simulink model "6DoF_V8_2024a_FULLY_WORKING_FG"  (R2024b)
settings: Solver=ode45  StartTime=0.0  StopTime=500  FixedStep=.01  MaxStep=.004  RelTol=1e-5  EnableMultiTasking=on
values from neighbouring files (symbols this model uses):
  ac = [0 0 0]    [Geom_6dof_V4_WITH_MAP.m]
  b = 33.4    [Geom_6dof_V4_WITH_MAP.m]
  bankrange = linspace(-pi,pi,100)    [Geom_6dof_V4_WITH_MAP.m]
  cbar = 5.7    [Geom_6dof_V4_WITH_MAP.m]
  cda2 = 0.33    [Geom_6dof_V4_WITH_MAP.m]
  cdo = 0.05    [Geom_6dof_V4_WITH_MAP.m]
  cg = [0 0 0]    [Geom_6dof_V4_WITH_MAP.m]
  cla = 4.44    [Geom_6dof_V4_WITH_MAP.m]
  cladot = 0    [Geom_6dof_V4_WITH_MAP.m]
  clb = -0.074    [Geom_6dof_V4_WITH_MAP.m]
  clda = -0.134    [Geom_6dof_V4_WITH_MAP.m]
  clde = 0.355    [Geom_6dof_V4_WITH_MAP.m]
  cldr = 0.107    [Geom_6dof_V4_WITH_MAP.m]
  clo = 0.41    [Geom_6dof_V4_WITH_MAP.m]
  clp = -0.410    (= -0.41)    [Geom_6dof_V4_WITH_MAP.m]
  clq = 3.8    [Geom_6dof_V4_WITH_MAP.m]
  clr = 0.107    [Geom_6dof_V4_WITH_MAP.m]
  cma = -0.683    [Geom_6dof_V4_WITH_MAP.m]
  cmadot = -4.36    [Geom_6dof_V4_WITH_MAP.m]
  cmde = -0.923    [Geom_6dof_V4_WITH_MAP.m]
  cmq = -9.96    [Geom_6dof_V4_WITH_MAP.m]
  cnb = 0.071    [Geom_6dof_V4_WITH_MAP.m]
  cnda = -0.0035    [Geom_6dof_V4_WITH_MAP.m]
  cndr = -0.072    [Geom_6dof_V4_WITH_MAP.m]
  cnp = -0.0575    [Geom_6dof_V4_WITH_MAP.m]
  cnr = -0.125    [Geom_6dof_V4_WITH_MAP.m]
  cyb = -0.564    [Geom_6dof_V4_WITH_MAP.m]
  cydr = 0.157    [Geom_6dof_V4_WITH_MAP.m]
  eng = [0 0 0]    [Geom_6dof_V4_WITH_MAP.m]
  initalt = 5000    [Geom_6dof_V4_WITH_MAP.m]
  initbank = 0    [Geom_6dof_V4_WITH_MAP.m]
  initeast = 0    [Geom_6dof_V4_WITH_MAP.m]
  inithead = 0    [Geom_6dof_V4_WITH_MAP.m]
  initnorth = 0    [Geom_6dof_V4_WITH_MAP.m]
  initp = 0    [Geom_6dof_V4_WITH_MAP.m]
  initpitch = initw/initu    (= -0.0287187462721)    [Geom_6dof_V4_WITH_MAP.m]
  initq = 0    [Geom_6dof_V4_WITH_MAP.m]
  initr = 0    [Geom_6dof_V4_WITH_MAP.m]
  initu = 226.333    [Geom_6dof_V4_WITH_MAP.m]
  initv = 0    [Geom_6dof_V4_WITH_MAP.m]
  initw = -6.5    [Geom_6dof_V4_WITH_MAP.m]
  jx = 1048    [Geom_6dof_V4_WITH_MAP.m]
  jxz = 0    [Geom_6dof_V4_WITH_MAP.m]
  jy = 3000    [Geom_6dof_V4_WITH_MAP.m]
  jz = 3500    [Geom_6dof_V4_WITH_MAP.m]
  sw = 184    [Geom_6dof_V4_WITH_MAP.m]
  weight = 2750    [Geom_6dof_V4_WITH_MAP.m]
  WP1 = [10000 10000 5000]    [Geom_6dof_V4_WITH_MAP.m]
  WP2 = [-10000 0 5500]    [Geom_6dof_V4_WITH_MAP.m]
  WP3 = [0 -10000 4500]    [Geom_6dof_V4_WITH_MAP.m]
libraries: slpidlib x10, simulink_extras x5, aerolibfltsims x2, aerolibanimutils x1, dspswit3 x1
(part 2 of 2)

== system 6DoF_V8_2024a_FULLY_WORKING_FG/Aircraft_Dynamics/Equations of motion numerical integration /Gravity Model ==
  Constant : Constant  Value=0
  Constant1 : Constant  Value=32.2
  Mux : Mux  Inputs=3
  Gravity : Outport
  wires:
  Constant/1 -> Mux/1, Mux/2
  Constant1/1 -> Mux/3
  Mux/1 -> Gravity/1

== system 6DoF_V8_2024a_FULLY_WORKING_FG/Aircraft_Dynamics/Equations of motion numerical integration /Inert-body ==
  Euler : Inport
  11 : Fcn  Expr=cos(u[2])*cos(u[3])
  12 : Fcn  Expr=-cos(u[1])*sin(u[3])+sin(u[1])*sin(u[2])*cos(u[3])
  13 : Fcn  Expr=sin(u[1])*sin(u[3])+cos(u[1])*sin(u[2])*cos(u[3])
  21 : Fcn  Expr=cos(u[2])*sin(u[3])
  22 : Fcn  Expr=cos(u[1])*cos(u[3]) + sin(u[1])*sin(u[2])*sin(u[3])
  23 : Fcn  Expr=-sin(u[1])*cos(u[3])+cos(u[1])*sin(u[2])*sin(u[3])
  31 : Fcn  Expr=-sin(u[2])
  32 : Fcn  Expr=sin(u[1]) * cos(u[2])
  33 : Fcn  Expr=cos(u[1])*cos(u[2])
  Matrix Concatenation : Concatenate  NumInputs=3  Mode=Multidimensional array
  Matrix Concatenation1 : Concatenate  NumInputs=3  Mode=Multidimensional array
  Matrix Concatenation2 : Concatenate  NumInputs=3  Mode=Multidimensional array
  Matrix Concatenation3 : Concatenate  NumInputs=3  Mode=Multidimensional array  ConcatenateDimension=2
  NEDtoBC : Outport
  wires:
  Euler/1 -> 11/1, 12/1, 13/1, 21/1, 22/1, 23/1, 31/1, 33/1, 32/1
  12/1 -> Matrix Concatenation/2
  11/1 -> Matrix Concatenation/1
  13/1 -> Matrix Concatenation/3
  22/1 -> Matrix Concatenation1/2
  21/1 -> Matrix Concatenation1/1
  23/1 -> Matrix Concatenation1/3
  32/1 -> Matrix Concatenation2/2
  31/1 -> Matrix Concatenation2/1
  33/1 -> Matrix Concatenation2/3
  Matrix Concatenation1/1 -> Matrix Concatenation3/2
  Matrix Concatenation/1 -> Matrix Concatenation3/1
  Matrix Concatenation2/1 -> Matrix Concatenation3/3
  Matrix Concatenation3/1 -> NEDtoBC/1

== system 6DoF_V8_2024a_FULLY_WORKING_FG/Aircraft_Dynamics/Equations of motion numerical integration /Kinematic Equiations ==
  note: 1  p
      | 2  q
      | 3  r
      | 4  bank
      | 5 pitch
      | 6 Yaw
  Rates : Inport
  2pi Bound : Subsystem  mask(2pi bound){}
      mask help: Bounds the input angle to [0, 2pi]. When 0 bound is exceeded the output wraps back to 2pi; when the 2pi bound is exceeded the output wraps back to 0.
      mask Help:
      | Bounds the input angle to [0, 2pi]. When 0 bound is exceeded the output wraps back to 2pi; when the 2pi bound is exceeded the output wraps back to 0.
      | <P><B>Input:</B> any angle in radians, from -Inf to Inf;</P>
      | <P><B>Output:</B> an angle in radians between zero and 2pi.</P>
  Demux : Demux  Outputs=3
      settings: DisplayOption=none
  Demux1 : Demux  Outputs=3
      settings: DisplayOption=none
  Demux2 : Demux  Outputs=3
      settings: DisplayOption=none
  Mux : Mux  Inputs=6
  Mux1 : Mux  Inputs=3
  Mux2 : Mux  Inputs=3
  Yaw rate : Fcn  Expr=(u[2] * sin(u[4]) + u[3] * cos(u[4]))/cos(u[5])
  bank : Integrator  InitialCondition=initbank
  heading : Integrator  InitialCondition=inithead
  pi Bound : Subsystem  mask(pi bound){}
      mask help: Bounds the input angle to [-pi, pi]. When -pi bound is exceeded the output wraps back to pi; when the pi bound is exceeded the output wraps back to -pi.
      mask Help:
      | Bounds the input angle to [-pi, pi]. When -pi bound is exceeded the output wraps back to pi; when the pi bound is exceeded the output wraps back to -pi.
      | <P><B>Input:</B> any angle in radians, from -Inf to Inf;</P>
      | <P><B>Output:</B> an angle in radians between -pi and pi.</P>
  pi Bound1 : Subsystem  mask(pi bound){}
      mask help: Bounds the input angle to [-pi, pi]. When -pi bound is exceeded the output wraps back to pi; when the pi bound is exceeded the output wraps back to -pi.
      mask Help:
      | Bounds the input angle to [-pi, pi]. When -pi bound is exceeded the output wraps back to pi; when the pi bound is exceeded the output wraps back to -pi.
      | <P><B>Input:</B> any angle in radians, from -Inf to Inf;</P>
      | <P><B>Output:</B> an angle in radians between -pi and pi.</P>
  pitch : Integrator  InitialCondition=initpitch
  pitch rate : Fcn  Expr=u[2] *cos(u[4]) - u[3] * sin(u[4])
  roll rate : Fcn  Expr=u[1] + tan(u[5])*(u[2]*sin(u[4])+u[3]*cos(u[4]))
  Euler angles : Outport
  wires:
  Rates/1 -> Demux/1
  Demux/2 -> Mux/2
  Demux/3 -> Mux/3
  Demux1/1 -> Mux/4
  Demux1/2 -> Mux/5
  Demux1/3 -> Mux/6
  Demux/1 -> Mux/1
  Mux/1 -> roll rate/1, Yaw rate/1, pitch rate/1
  Demux2/3 -> 2pi Bound/1(In)
  Demux2/2 -> pi Bound/1(In)
  Demux2/1 -> pi Bound1/1(In)
  Mux2/1 -> Euler angles/1
  pi Bound/1(Out) -> Mux2/2
  pi Bound1/1(Out) -> Mux2/1
  2pi Bound/1(Out) -> Mux2/3
  pitch rate/1 -> pitch/1
  roll rate/1 -> bank/1
  Yaw rate/1 -> heading/1
  bank/1 -> Mux1/1
  pitch/1 -> Mux1/2
  heading/1 -> Mux1/3
  Mux1/1 -> Demux2/1, Demux1/1

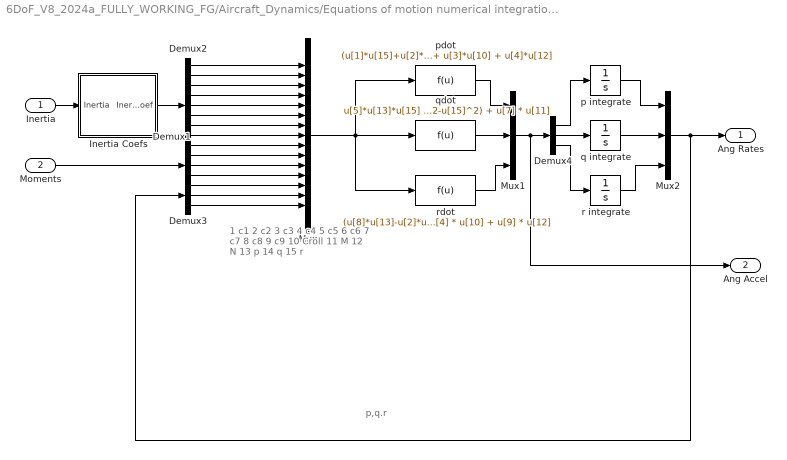
== system 6DoF_V8_2024a_FULLY_WORKING_FG/Aircraft_Dynamics/Equations of motion numerical integration /Moment Equations ==
  note: 1   c1
      | 2   c2
      | 3   c3
      | 4  c4
      | 5  c5
      | 6  c6
      | 7  c7
      | 8  c8
      | 9  c9
      | 10 Croll
      | 11  M
      | 12  N
      | 13  p
      | 14  q
      | 15  r
  note: p,q.r
  Inertia : Inport
  Moments : Inport  Port=2
  Demux1 : Demux  Outputs=3
      settings: DisplayOption=none
  Demux2 : Demux  Outputs=9
      settings: DisplayOption=none
  Demux3 : Demux  Outputs=3
      settings: DisplayOption=none
  Demux4 : Demux  Outputs=3
      settings: DisplayOption=none
  Inertia Coefs : Subsystem
  Mux : Mux  Inputs=15
  Mux1 : Mux  Inputs=3
  Mux2 : Mux  Inputs=3
  p integrate : Integrator  InitialCondition=initp
  pdot : Fcn  Expr=(u[1]*u[15]+u[2]*u[13])*u[14] + u[3]*u[10] + u[4]*u[12]
  q integrate : Integrator  InitialCondition=initq
  qdot : Fcn  Expr=u[5]*u[13]*u[15] - u[6]*(u[13]^2-u[15]^2) + u[7] * u[11]
  r integrate : Integrator  InitialCondition=initr
  rdot : Fcn  Expr=(u[8]*u[13]-u[2]*u[15]) * u[14] + u[4] * u[10] + u[9] * u[12]
  Ang Rates : Outport
  Ang Accel : Outport  Port=2
  wires:
  Inertia/1 -> Inertia Coefs/1(Inertia)
  Moments/1 -> Demux1/1
  Inertia Coefs/1(Iner Coef) -> Demux2/1
  Demux2/1 -> Mux/1
  Demux2/2 -> Mux/2
  Demux2/3 -> Mux/3
  Demux2/4 -> Mux/4
  Demux2/5 -> Mux/5
  Demux2/6 -> Mux/6
  Demux2/7 -> Mux/7
  Demux2/8 -> Mux/8
  Demux2/9 -> Mux/9
  Demux1/1 -> Mux/10
  Demux1/2 -> Mux/11
  Demux1/3 -> Mux/12
  Demux3/1 -> Mux/13
  Demux3/2 -> Mux/14
  Demux3/3 -> Mux/15
  Mux/1 -> pdot/1, qdot/1, rdot/1
  qdot/1 -> Mux1/2
  pdot/1 -> Mux1/1
  rdot/1 -> Mux1/3
  Mux1/1 -> Ang Accel/1, Demux4/1
  Demux4/1 -> p integrate/1
  Demux4/2 -> q integrate/1
  Demux4/3 -> r integrate/1
  Mux2/1 -> Ang Rates/1, Demux3/1
  p integrate/1 -> Mux2/1
  q integrate/1 -> Mux2/2
  r integrate/1 -> Mux2/3

== system 6DoF_V8_2024a_FULLY_WORKING_FG/Aircraft_Dynamics/Linear Acc and Moments/Cross Prod Moment due Leng ==
  Vec 1 : Inport
  Vec 2 : Inport  Port=2
  Check prob not zero : Constant  Value=0
  Demux : Demux  Outputs=3
      settings: DisplayOption=none
  J axis : Fcn  Expr=u[4]*u[3] - u[6]*u[1]
  Mux : Mux  Inputs=6
  Mux1 : Mux  Inputs=3
  i axis : Fcn  Expr=u[6]*u[2] - u[5]*u[3]
  k axis : Fcn  Expr=u[5]*u[1] - u[4]*u[2]
  X Prod : Outport
  wires:
  Vec 2/1 -> Mux/4
  Vec 1/1 -> Demux/1
  Demux/1 -> Mux/1
  Check prob not zero/1 -> Mux/5, Mux/6
  Demux/3 -> Mux/3
  Demux/2 -> Mux/2
  Mux/1 -> i axis/1, J axis/1, k axis/1
  J axis/1 -> Mux1/2
  i axis/1 -> Mux1/1
  k axis/1 -> Mux1/3
  Mux1/1 -> X Prod/1

== system 6DoF_V8_2024a_FULLY_WORKING_FG/Aircraft_Dynamics/Linear Acc and Moments/Cross Prod Moment due to Aero ==
  Vec 1 : Inport
  Vec 2 : Inport  Port=2
  Demux : Demux  Outputs=3
      settings: DisplayOption=none
  Demux1 : Demux  Outputs=3
      settings: DisplayOption=none
  J axis : Fcn  Expr=u[4]*u[3] - u[6]*u[1]
  Mux : Mux  Inputs=6
  Mux1 : Mux  Inputs=3
  i axis : Fcn  Expr=u[6]*u[2] - u[5]*u[3]
  k axis : Fcn  Expr=u[5]*u[1] - u[4]*u[2]
  X Prod : Outport
  wires:
  Vec 2/1 -> Demux1/1
  Vec 1/1 -> Demux/1
  Demux/1 -> Mux/1
  Demux1/3 -> Mux/6
  Demux1/2 -> Mux/5
  Demux1/1 -> Mux/4
  Demux/3 -> Mux/3
  Demux/2 -> Mux/2
  Mux/1 -> i axis/1, J axis/1, k axis/1
  J axis/1 -> Mux1/2
  i axis/1 -> Mux1/1
  k axis/1 -> Mux1/3
  Mux1/1 -> X Prod/1

== system 6DoF_V8_2024a_FULLY_WORKING_FG/Waypoint Calc/Altitude Hold Autopilot/Climb ==
  R/C : Inport
  Action Port : ActionPort  ActionPortLabel=if(u1 < -100)
  PID Controller : slpidlib/PID Controller  Controller=PI  Form=Parallel  TimeDomain=Continuous-time  UseExternalTs=off  SampleTime=-1  IntegratorMethod=Forward Euler  FilterMethod=Forward Euler  ControllerParametersSource=internal  P=-9.44462319155585e-06  I=-9.44462319155585e-06  UseKiTs=off  D=0  UseExternalDerivativeSource=off  N=100  UseFilter=on  TunerSelectOption=Transfer Function Based (PID Tuner App)  InitialConditionSource=internal  InitialConditionForIntegrator=0  InitialConditionForFilter=0  DifferentiatorICPrevScaledInput=0  ExternalReset=none  TrackingMode=off  Kt=1  LimitOutput=off  SatLimitsSource=internal  UpperSaturationLimit=inf  LowerSaturationLimit=-inf  LinearizeAsGain=on  AntiWindupMode=none  Kb=1  LimitIntegrator=off  UpperIntegratorSaturationLimit=inf  LowerIntegratorSaturationLimit=-inf  POutMin=[]  POutMax=[]  IOutMin=[]  IOutMax=[]  DOutMin=[]  DOutMax=[]  NOutMin=[]  NOutMax=[]  SumOutMin=[]  SumOutMax=[]  SaturationOutMin=[]  SaturationOutMax=[]  PParamMin=[]  PParamMax=[]  IParamMin=[]  IParamMax=[]  DParamMin=[]  DParamMax=[]  NParamMin=[]  NParamMax=[]  KbParamMin=[]  KbParamMax=[]  KtParamMin=[]  KtParamMax=[]  KbOutMin=[]  KbOutMax=[]  KtOutMin=[]  KtOutMax=[]  IntegratorOutMin=[]  IntegratorOutMax=[]  FilterOutMin=[]  FilterOutMax=[]  SumI1OutMin=[]  SumI1OutMax=[]  SumI2OutMin=[]  SumI2OutMax=[]  SumI3OutMin=[]  SumI3OutMax=[]  SumI4OutMin=[]  SumI4OutMax=[]  SumDOutMin=[]  SumDOutMax=[]  DifferentiatorOutMin=[]  DifferentiatorOutMax=[]  FilterDiffOutCoefMin=[]  FilterDiffOutCoefMax=[]  ReciprocalOutMin=[]  ReciprocalOutMax=[]  SumDenOutMin=[]  SumDenOutMax=[]  SumNumOutMin=[]  SumNumOutMax=[]  DivideOutMin=[]  DivideOutMax=[]  UdiffTsProdOutMin=[]  UdiffTsProdOutMax=[]  NTsProdOutMin=[]  NTsProdOutMax=[]  UintegralTsProdOutMin=[]  UintegralTsProdOutMax=[]  UngainTsProdOutMin=[]  UngainTsProdOutMax=[]  ClampingZeroOutDataTypeStr=Inherit: Inherit via back propagation  ClampingZeroOutMin=[]  ClampingZeroOutMax=[]  FilterDenConstantOutDataTypeStr=Inherit: Inherit via back propagation  FilterDenConstantOutMin=[]  FilterDenConstantOutMax=[]  PCopyOutDataTypeStr=Inherit: Inherit via back propagation  PCopyOutMin=[]  PCopyOutMax=[]  NCopyOutDataTypeStr=Inherit: Inherit via back propagation  NCopyOutMin=[]  NCopyOutMax=[]  IntegratorContinuousStateAttributes=''  IntegratorStateMustResolveToSignalObject=off  IntegratorRTWStateStorageClass=Auto  FilterContinuousStateAttributes=''  FilterStateMustResolveToSignalObject=off  FilterRTWStateStorageClass=Auto  ParallelPVariant=InternalParameters  IdealPVariant=Disabled  IVariant=InternalParameters  DVariant=Disabled  IntegratorVariant=Continuous  SatVariant=Disabled  AWVariant=Passthrough  PCopyVariant=Disabled  TRVariant=Disabled  FdbkBlocksVariant=Forward  IdealPFdbkVariant=Disabled  SatFdbkVariant=Disabled  DerivativeFilterVariant=Disabled  NVariant=Disabled  NCopyVariant=Disabled_SignalSpec  FilterICVariant=Disabled  IntegratorICVariant=InternalICs  ExternalResetVariant=Disabled  TRSumVariant=Passthrough  SumFdbkVariant=Disabled  SumVariant=Sum_PI  TsampFilterVariant=InternalTs  TsampNgainVariant=Passthrough  TsampIntegralVariant=Disabled_SignalSpec  ExternalSaturationOutDataTypeStr=Inherit: Same as second input  DerivativeSourceVariant=Disabled  PreIntVariant=InternalPreInt
  PID Controller1 : slpidlib/PID Controller  Controller=PI  Form=Parallel  TimeDomain=Continuous-time  UseExternalTs=off  SampleTime=-1  IntegratorMethod=Forward Euler  FilterMethod=Forward Euler  ControllerParametersSource=internal  P=-0.000713863552295223  I=-0.000143178740792475  UseKiTs=off  D=0  UseExternalDerivativeSource=off  N=100  UseFilter=on  TunerSelectOption=Transfer Function Based (PID Tuner App)  InitialConditionSource=internal  InitialConditionForIntegrator=0  InitialConditionForFilter=0  DifferentiatorICPrevScaledInput=0  ExternalReset=none  TrackingMode=off  Kt=1  LimitOutput=off  SatLimitsSource=internal  UpperSaturationLimit=inf  LowerSaturationLimit=-inf  LinearizeAsGain=on  AntiWindupMode=none  Kb=1  LimitIntegrator=off  UpperIntegratorSaturationLimit=inf  LowerIntegratorSaturationLimit=-inf  POutMin=[]  POutMax=[]  IOutMin=[]  IOutMax=[]  DOutMin=[]  DOutMax=[]  NOutMin=[]  NOutMax=[]  SumOutMin=[]  SumOutMax=[]  SaturationOutMin=[]  SaturationOutMax=[]  PParamMin=[]  PParamMax=[]  IParamMin=[]  IParamMax=[]  DParamMin=[]  DParamMax=[]  NParamMin=[]  NParamMax=[]  KbParamMin=[]  KbParamMax=[]  KtParamMin=[]  KtParamMax=[]  KbOutMin=[]  KbOutMax=[]  KtOutMin=[]  KtOutMax=[]  IntegratorOutMin=[]  IntegratorOutMax=[]  FilterOutMin=[]  FilterOutMax=[]  SumI1OutMin=[]  SumI1OutMax=[]  SumI2OutMin=[]  SumI2OutMax=[]  SumI3OutMin=[]  SumI3OutMax=[]  SumI4OutMin=[]  SumI4OutMax=[]  SumDOutMin=[]  SumDOutMax=[]  DifferentiatorOutMin=[]  DifferentiatorOutMax=[]  FilterDiffOutCoefMin=[]  FilterDiffOutCoefMax=[]  ReciprocalOutMin=[]  ReciprocalOutMax=[]  SumDenOutMin=[]  SumDenOutMax=[]  SumNumOutMin=[]  SumNumOutMax=[]  DivideOutMin=[]  DivideOutMax=[]  UdiffTsProdOutMin=[]  UdiffTsProdOutMax=[]  NTsProdOutMin=[]  NTsProdOutMax=[]  UintegralTsProdOutMin=[]  UintegralTsProdOutMax=[]  UngainTsProdOutMin=[]  UngainTsProdOutMax=[]  ClampingZeroOutDataTypeStr=Inherit: Inherit via back propagation  ClampingZeroOutMin=[]  ClampingZeroOutMax=[]  FilterDenConstantOutDataTypeStr=Inherit: Inherit via back propagation  FilterDenConstantOutMin=[]  FilterDenConstantOutMax=[]  PCopyOutDataTypeStr=Inherit: Inherit via back propagation  PCopyOutMin=[]  PCopyOutMax=[]  NCopyOutDataTypeStr=Inherit: Inherit via back propagation  NCopyOutMin=[]  NCopyOutMax=[]  IntegratorContinuousStateAttributes=''  IntegratorStateMustResolveToSignalObject=off  IntegratorRTWStateStorageClass=Auto  FilterContinuousStateAttributes=''  FilterStateMustResolveToSignalObject=off  FilterRTWStateStorageClass=Auto  ParallelPVariant=InternalParameters  IdealPVariant=Disabled  IVariant=InternalParameters  DVariant=Disabled  IntegratorVariant=Continuous  SatVariant=Disabled  AWVariant=Passthrough  PCopyVariant=Disabled  TRVariant=Disabled  FdbkBlocksVariant=Forward  IdealPFdbkVariant=Disabled  SatFdbkVariant=Disabled  DerivativeFilterVariant=Disabled  NVariant=Disabled  NCopyVariant=Disabled_SignalSpec  FilterICVariant=Disabled  IntegratorICVariant=InternalICs  ExternalResetVariant=Disabled  TRSumVariant=Passthrough  SumFdbkVariant=Disabled  SumVariant=Sum_PI  TsampFilterVariant=InternalTs  TsampNgainVariant=Passthrough  TsampIntegralVariant=Disabled_SignalSpec  ExternalSaturationOutDataTypeStr=Inherit: Same as second input  DerivativeSourceVariant=Disabled  PreIntVariant=InternalPreInt
  R/C_CMD : Constant  Value=12
  R/C_CMD1 : Constant
  Sum : Sum  Inputs=|+-
  del_e : Outport
  Debug : Outport  Port=2
  wires:
  R/C/1 -> Sum/1
  R/C_CMD/1 -> Sum/2
  R/C_CMD1/1 -> Debug/1
  Sum/1 -> PID Controller1/1
  PID Controller1/1 -> del_e/1

== system 6DoF_V8_2024a_FULLY_WORKING_FG/Waypoint Calc/Altitude Hold Autopilot/Descent ==
  R/C : Inport
  Action Port : ActionPort  ActionPortLabel=elseif(u1 > 100)
  Gain : Gain
  PID Controller : slpidlib/PID Controller  Controller=PI  Form=Parallel  TimeDomain=Continuous-time  UseExternalTs=off  SampleTime=-1  IntegratorMethod=Forward Euler  FilterMethod=Forward Euler  ControllerParametersSource=internal  P=-9.44462319155585e-06  I=-9.44462319155585e-06  UseKiTs=off  D=0  UseExternalDerivativeSource=off  N=100  UseFilter=on  TunerSelectOption=Transfer Function Based (PID Tuner App)  InitialConditionSource=internal  InitialConditionForIntegrator=0  InitialConditionForFilter=0  DifferentiatorICPrevScaledInput=0  ExternalReset=none  TrackingMode=off  Kt=1  LimitOutput=off  SatLimitsSource=internal  UpperSaturationLimit=inf  LowerSaturationLimit=-inf  LinearizeAsGain=on  AntiWindupMode=none  Kb=1  LimitIntegrator=off  UpperIntegratorSaturationLimit=inf  LowerIntegratorSaturationLimit=-inf  POutMin=[]  POutMax=[]  IOutMin=[]  IOutMax=[]  DOutMin=[]  DOutMax=[]  NOutMin=[]  NOutMax=[]  SumOutMin=[]  SumOutMax=[]  SaturationOutMin=[]  SaturationOutMax=[]  PParamMin=[]  PParamMax=[]  IParamMin=[]  IParamMax=[]  DParamMin=[]  DParamMax=[]  NParamMin=[]  NParamMax=[]  KbParamMin=[]  KbParamMax=[]  KtParamMin=[]  KtParamMax=[]  KbOutMin=[]  KbOutMax=[]  KtOutMin=[]  KtOutMax=[]  IntegratorOutMin=[]  IntegratorOutMax=[]  FilterOutMin=[]  FilterOutMax=[]  SumI1OutMin=[]  SumI1OutMax=[]  SumI2OutMin=[]  SumI2OutMax=[]  SumI3OutMin=[]  SumI3OutMax=[]  SumI4OutMin=[]  SumI4OutMax=[]  SumDOutMin=[]  SumDOutMax=[]  DifferentiatorOutMin=[]  DifferentiatorOutMax=[]  FilterDiffOutCoefMin=[]  FilterDiffOutCoefMax=[]  ReciprocalOutMin=[]  ReciprocalOutMax=[]  SumDenOutMin=[]  SumDenOutMax=[]  SumNumOutMin=[]  SumNumOutMax=[]  DivideOutMin=[]  DivideOutMax=[]  UdiffTsProdOutMin=[]  UdiffTsProdOutMax=[]  NTsProdOutMin=[]  NTsProdOutMax=[]  UintegralTsProdOutMin=[]  UintegralTsProdOutMax=[]  UngainTsProdOutMin=[]  UngainTsProdOutMax=[]  ClampingZeroOutDataTypeStr=Inherit: Inherit via back propagation  ClampingZeroOutMin=[]  ClampingZeroOutMax=[]  FilterDenConstantOutDataTypeStr=Inherit: Inherit via back propagation  FilterDenConstantOutMin=[]  FilterDenConstantOutMax=[]  PCopyOutDataTypeStr=Inherit: Inherit via back propagation  PCopyOutMin=[]  PCopyOutMax=[]  NCopyOutDataTypeStr=Inherit: Inherit via back propagation  NCopyOutMin=[]  NCopyOutMax=[]  IntegratorContinuousStateAttributes=''  IntegratorStateMustResolveToSignalObject=off  IntegratorRTWStateStorageClass=Auto  FilterContinuousStateAttributes=''  FilterStateMustResolveToSignalObject=off  FilterRTWStateStorageClass=Auto  ParallelPVariant=InternalParameters  IdealPVariant=Disabled  IVariant=InternalParameters  DVariant=Disabled  IntegratorVariant=Continuous  SatVariant=Disabled  AWVariant=Passthrough  PCopyVariant=Disabled  TRVariant=Disabled  FdbkBlocksVariant=Forward  IdealPFdbkVariant=Disabled  SatFdbkVariant=Disabled  DerivativeFilterVariant=Disabled  NVariant=Disabled  NCopyVariant=Disabled_SignalSpec  FilterICVariant=Disabled  IntegratorICVariant=InternalICs  ExternalResetVariant=Disabled  TRSumVariant=Passthrough  SumFdbkVariant=Disabled  SumVariant=Sum_PI  TsampFilterVariant=InternalTs  TsampNgainVariant=Passthrough  TsampIntegralVariant=Disabled_SignalSpec  ExternalSaturationOutDataTypeStr=Inherit: Same as second input  DerivativeSourceVariant=Disabled  PreIntVariant=InternalPreInt
  PID Controller1 : slpidlib/PID Controller  Controller=PI  Form=Parallel  TimeDomain=Continuous-time  UseExternalTs=off  SampleTime=-1  IntegratorMethod=Forward Euler  FilterMethod=Forward Euler  ControllerParametersSource=internal  P=-0.000713863552295223  I=-0.000143178740792475  UseKiTs=off  D=0  UseExternalDerivativeSource=off  N=100  UseFilter=on  TunerSelectOption=Transfer Function Based (PID Tuner App)  InitialConditionSource=internal  InitialConditionForIntegrator=0  InitialConditionForFilter=0  DifferentiatorICPrevScaledInput=0  ExternalReset=none  TrackingMode=off  Kt=1  LimitOutput=off  SatLimitsSource=internal  UpperSaturationLimit=inf  LowerSaturationLimit=-inf  LinearizeAsGain=on  AntiWindupMode=none  Kb=1  LimitIntegrator=off  UpperIntegratorSaturationLimit=inf  LowerIntegratorSaturationLimit=-inf  POutMin=[]  POutMax=[]  IOutMin=[]  IOutMax=[]  DOutMin=[]  DOutMax=[]  NOutMin=[]  NOutMax=[]  SumOutMin=[]  SumOutMax=[]  SaturationOutMin=[]  SaturationOutMax=[]  PParamMin=[]  PParamMax=[]  IParamMin=[]  IParamMax=[]  DParamMin=[]  DParamMax=[]  NParamMin=[]  NParamMax=[]  KbParamMin=[]  KbParamMax=[]  KtParamMin=[]  KtParamMax=[]  KbOutMin=[]  KbOutMax=[]  KtOutMin=[]  KtOutMax=[]  IntegratorOutMin=[]  IntegratorOutMax=[]  FilterOutMin=[]  FilterOutMax=[]  SumI1OutMin=[]  SumI1OutMax=[]  SumI2OutMin=[]  SumI2OutMax=[]  SumI3OutMin=[]  SumI3OutMax=[]  SumI4OutMin=[]  SumI4OutMax=[]  SumDOutMin=[]  SumDOutMax=[]  DifferentiatorOutMin=[]  DifferentiatorOutMax=[]  FilterDiffOutCoefMin=[]  FilterDiffOutCoefMax=[]  ReciprocalOutMin=[]  ReciprocalOutMax=[]  SumDenOutMin=[]  SumDenOutMax=[]  SumNumOutMin=[]  SumNumOutMax=[]  DivideOutMin=[]  DivideOutMax=[]  UdiffTsProdOutMin=[]  UdiffTsProdOutMax=[]  NTsProdOutMin=[]  NTsProdOutMax=[]  UintegralTsProdOutMin=[]  UintegralTsProdOutMax=[]  UngainTsProdOutMin=[]  UngainTsProdOutMax=[]  ClampingZeroOutDataTypeStr=Inherit: Inherit via back propagation  ClampingZeroOutMin=[]  ClampingZeroOutMax=[]  FilterDenConstantOutDataTypeStr=Inherit: Inherit via back propagation  FilterDenConstantOutMin=[]  FilterDenConstantOutMax=[]  PCopyOutDataTypeStr=Inherit: Inherit via back propagation  PCopyOutMin=[]  PCopyOutMax=[]  NCopyOutDataTypeStr=Inherit: Inherit via back propagation  NCopyOutMin=[]  NCopyOutMax=[]  IntegratorContinuousStateAttributes=''  IntegratorStateMustResolveToSignalObject=off  IntegratorRTWStateStorageClass=Auto  FilterContinuousStateAttributes=''  FilterStateMustResolveToSignalObject=off  FilterRTWStateStorageClass=Auto  ParallelPVariant=InternalParameters  IdealPVariant=Disabled  IVariant=InternalParameters  DVariant=Disabled  IntegratorVariant=Continuous  SatVariant=Disabled  AWVariant=Passthrough  PCopyVariant=Disabled  TRVariant=Disabled  FdbkBlocksVariant=Forward  IdealPFdbkVariant=Disabled  SatFdbkVariant=Disabled  DerivativeFilterVariant=Disabled  NVariant=Disabled  NCopyVariant=Disabled_SignalSpec  FilterICVariant=Disabled  IntegratorICVariant=InternalICs  ExternalResetVariant=Disabled  TRSumVariant=Passthrough  SumFdbkVariant=Disabled  SumVariant=Sum_PI  TsampFilterVariant=InternalTs  TsampNgainVariant=Passthrough  TsampIntegralVariant=Disabled_SignalSpec  ExternalSaturationOutDataTypeStr=Inherit: Same as second input  DerivativeSourceVariant=Disabled  PreIntVariant=InternalPreInt
  R/C_CMD : Constant  Value=-12
  R/C_CMD1 : Constant  Value=2
  Sum : Sum  Inputs=|+-
  del_e : Outport
  Debug : Outport  Port=2
  wires:
  R/C_CMD1/1 -> Debug/1
  R/C/1 -> Sum/1
  R/C_CMD/1 -> Sum/2
  Gain/1 -> del_e/1
  Sum/1 -> PID Controller1/1
  PID Controller1/1 -> Gain/1

== system 6DoF_V8_2024a_FULLY_WORKING_FG/Waypoint Calc/Altitude Hold Autopilot/Level ==
  h_error : Inport
  Action Port : ActionPort  ActionPortLabel=else
  Constant : Constant  Value=3
  ORIG : slpidlib/PID Controller  Controller=PI  Form=Parallel  TimeDomain=Continuous-time  UseExternalTs=off  SampleTime=-1  IntegratorMethod=Forward Euler  FilterMethod=Forward Euler  ControllerParametersSource=internal  P=-1.24283450149489e-05  I=-6.32459130011013e-08  UseKiTs=off  D=0  UseExternalDerivativeSource=off  N=100  UseFilter=on  TunerSelectOption=Transfer Function Based (PID Tuner App)  InitialConditionSource=internal  InitialConditionForIntegrator=0  InitialConditionForFilter=0  DifferentiatorICPrevScaledInput=0  ExternalReset=none  TrackingMode=off  Kt=1  LimitOutput=off  SatLimitsSource=internal  UpperSaturationLimit=inf  LowerSaturationLimit=-inf  LinearizeAsGain=on  AntiWindupMode=none  Kb=1  LimitIntegrator=off  UpperIntegratorSaturationLimit=inf  LowerIntegratorSaturationLimit=-inf  POutMin=[]  POutMax=[]  IOutMin=[]  IOutMax=[]  DOutMin=[]  DOutMax=[]  NOutMin=[]  NOutMax=[]  SumOutMin=[]  SumOutMax=[]  SaturationOutMin=[]  SaturationOutMax=[]  PParamMin=[]  PParamMax=[]  IParamMin=[]  IParamMax=[]  DParamMin=[]  DParamMax=[]  NParamMin=[]  NParamMax=[]  KbParamMin=[]  KbParamMax=[]  KtParamMin=[]  KtParamMax=[]  KbOutMin=[]  KbOutMax=[]  KtOutMin=[]  KtOutMax=[]  IntegratorOutMin=[]  IntegratorOutMax=[]  FilterOutMin=[]  FilterOutMax=[]  SumI1OutMin=[]  SumI1OutMax=[]  SumI2OutMin=[]  SumI2OutMax=[]  SumI3OutMin=[]  SumI3OutMax=[]  SumI4OutMin=[]  SumI4OutMax=[]  SumDOutMin=[]  SumDOutMax=[]  DifferentiatorOutMin=[]  DifferentiatorOutMax=[]  FilterDiffOutCoefMin=[]  FilterDiffOutCoefMax=[]  ReciprocalOutMin=[]  ReciprocalOutMax=[]  SumDenOutMin=[]  SumDenOutMax=[]  SumNumOutMin=[]  SumNumOutMax=[]  DivideOutMin=[]  DivideOutMax=[]  UdiffTsProdOutMin=[]  UdiffTsProdOutMax=[]  NTsProdOutMin=[]  NTsProdOutMax=[]  UintegralTsProdOutMin=[]  UintegralTsProdOutMax=[]  UngainTsProdOutMin=[]  UngainTsProdOutMax=[]  ClampingZeroOutDataTypeStr=Inherit: Inherit via back propagation  ClampingZeroOutMin=[]  ClampingZeroOutMax=[]  FilterDenConstantOutDataTypeStr=Inherit: Inherit via back propagation  FilterDenConstantOutMin=[]  FilterDenConstantOutMax=[]  PCopyOutDataTypeStr=Inherit: Inherit via back propagation  PCopyOutMin=[]  PCopyOutMax=[]  NCopyOutDataTypeStr=Inherit: Inherit via back propagation  NCopyOutMin=[]  NCopyOutMax=[]  IntegratorContinuousStateAttributes=''  IntegratorStateMustResolveToSignalObject=off  IntegratorRTWStateStorageClass=Auto  FilterContinuousStateAttributes=''  FilterStateMustResolveToSignalObject=off  FilterRTWStateStorageClass=Auto  ParallelPVariant=InternalParameters  IdealPVariant=Disabled  IVariant=InternalParameters  DVariant=Disabled  IntegratorVariant=Continuous  SatVariant=Disabled  AWVariant=Passthrough  PCopyVariant=Disabled  TRVariant=Disabled  FdbkBlocksVariant=Forward  IdealPFdbkVariant=Disabled  SatFdbkVariant=Disabled  DerivativeFilterVariant=Disabled  NVariant=Disabled  NCopyVariant=Disabled_SignalSpec  FilterICVariant=Disabled  IntegratorICVariant=InternalICs  ExternalResetVariant=Disabled  TRSumVariant=Passthrough  SumFdbkVariant=Disabled  SumVariant=Sum_PI  TsampFilterVariant=InternalTs  TsampNgainVariant=Passthrough  TsampIntegralVariant=Disabled_SignalSpec  ExternalSaturationOutDataTypeStr=Inherit: Same as second input  DerivativeSourceVariant=Disabled  PreIntVariant=InternalPreInt
  Try 1 : slpidlib/PID Controller  Controller=PI  Form=Parallel  TimeDomain=Continuous-time  UseExternalTs=off  SampleTime=-1  IntegratorMethod=Forward Euler  FilterMethod=Forward Euler  ControllerParametersSource=internal  P=-1.56673325043759e-04 *0.8  I=-1.17894403069236e-06  UseKiTs=off  D=0  UseExternalDerivativeSource=off  N=100  UseFilter=on  TunerSelectOption=Transfer Function Based (PID Tuner App)  InitialConditionSource=internal  InitialConditionForIntegrator=0  InitialConditionForFilter=0  DifferentiatorICPrevScaledInput=0  ExternalReset=none  TrackingMode=off  Kt=1  LimitOutput=off  SatLimitsSource=internal  UpperSaturationLimit=inf  LowerSaturationLimit=-inf  LinearizeAsGain=on  AntiWindupMode=none  Kb=1  LimitIntegrator=off  UpperIntegratorSaturationLimit=inf  LowerIntegratorSaturationLimit=-inf  POutMin=[]  POutMax=[]  IOutMin=[]  IOutMax=[]  DOutMin=[]  DOutMax=[]  NOutMin=[]  NOutMax=[]  SumOutMin=[]  SumOutMax=[]  SaturationOutMin=[]  SaturationOutMax=[]  PParamMin=[]  PParamMax=[]  IParamMin=[]  IParamMax=[]  DParamMin=[]  DParamMax=[]  NParamMin=[]  NParamMax=[]  KbParamMin=[]  KbParamMax=[]  KtParamMin=[]  KtParamMax=[]  KbOutMin=[]  KbOutMax=[]  KtOutMin=[]  KtOutMax=[]  IntegratorOutMin=[]  IntegratorOutMax=[]  FilterOutMin=[]  FilterOutMax=[]  SumI1OutMin=[]  SumI1OutMax=[]  SumI2OutMin=[]  SumI2OutMax=[]  SumI3OutMin=[]  SumI3OutMax=[]  SumI4OutMin=[]  SumI4OutMax=[]  SumDOutMin=[]  SumDOutMax=[]  DifferentiatorOutMin=[]  DifferentiatorOutMax=[]  FilterDiffOutCoefMin=[]  FilterDiffOutCoefMax=[]  ReciprocalOutMin=[]  ReciprocalOutMax=[]  SumDenOutMin=[]  SumDenOutMax=[]  SumNumOutMin=[]  SumNumOutMax=[]  DivideOutMin=[]  DivideOutMax=[]  UdiffTsProdOutMin=[]  UdiffTsProdOutMax=[]  NTsProdOutMin=[]  NTsProdOutMax=[]  UintegralTsProdOutMin=[]  UintegralTsProdOutMax=[]  UngainTsProdOutMin=[]  UngainTsProdOutMax=[]  ClampingZeroOutDataTypeStr=Inherit: Inherit via back propagation  ClampingZeroOutMin=[]  ClampingZeroOutMax=[]  FilterDenConstantOutDataTypeStr=Inherit: Inherit via back propagation  FilterDenConstantOutMin=[]  FilterDenConstantOutMax=[]  PCopyOutDataTypeStr=Inherit: Inherit via back propagation  PCopyOutMin=[]  PCopyOutMax=[]  NCopyOutDataTypeStr=Inherit: Inherit via back propagation  NCopyOutMin=[]  NCopyOutMax=[]  IntegratorContinuousStateAttributes=''  IntegratorStateMustResolveToSignalObject=off  IntegratorRTWStateStorageClass=Auto  FilterContinuousStateAttributes=''  FilterStateMustResolveToSignalObject=off  FilterRTWStateStorageClass=Auto  ParallelPVariant=InternalParameters  IdealPVariant=Disabled  IVariant=InternalParameters  DVariant=Disabled  IntegratorVariant=Continuous  SatVariant=Disabled  AWVariant=Passthrough  PCopyVariant=Disabled  TRVariant=Disabled  FdbkBlocksVariant=Forward  IdealPFdbkVariant=Disabled  SatFdbkVariant=Disabled  DerivativeFilterVariant=Disabled  NVariant=Disabled  NCopyVariant=Disabled_SignalSpec  FilterICVariant=Disabled  IntegratorICVariant=InternalICs  ExternalResetVariant=Disabled  TRSumVariant=Passthrough  SumFdbkVariant=Disabled  SumVariant=Sum_PI  TsampFilterVariant=InternalTs  TsampNgainVariant=Passthrough  TsampIntegralVariant=Disabled_SignalSpec  ExternalSaturationOutDataTypeStr=Inherit: Same as second input  DerivativeSourceVariant=Disabled  PreIntVariant=InternalPreInt
  Try 2 : slpidlib/PID Controller  Controller=PID  Form=Parallel  TimeDomain=Continuous-time  UseExternalTs=off  SampleTime=-1  IntegratorMethod=Forward Euler  FilterMethod=Forward Euler  ControllerParametersSource=internal  P=-1.82540369611787e-05  I=-2.94497758926846e-07  UseKiTs=off  D=-0.00015961532293143  UseExternalDerivativeSource=off  N=22.9108316729658  UseFilter=on  TunerSelectOption=Transfer Function Based (PID Tuner App)  InitialConditionSource=internal  InitialConditionForIntegrator=0  InitialConditionForFilter=0  DifferentiatorICPrevScaledInput=0  ExternalReset=none  TrackingMode=off  Kt=1  LimitOutput=off  SatLimitsSource=internal  UpperSaturationLimit=inf  LowerSaturationLimit=-inf  LinearizeAsGain=on  AntiWindupMode=none  Kb=1  LimitIntegrator=off  UpperIntegratorSaturationLimit=inf  LowerIntegratorSaturationLimit=-inf  POutMin=[]  POutMax=[]  IOutMin=[]  IOutMax=[]  DOutMin=[]  DOutMax=[]  NOutMin=[]  NOutMax=[]  SumOutMin=[]  SumOutMax=[]  SaturationOutMin=[]  SaturationOutMax=[]  PParamMin=[]  PParamMax=[]  IParamMin=[]  IParamMax=[]  DParamMin=[]  DParamMax=[]  NParamMin=[]  NParamMax=[]  KbParamMin=[]  KbParamMax=[]  KtParamMin=[]  KtParamMax=[]  KbOutMin=[]  KbOutMax=[]  KtOutMin=[]  KtOutMax=[]  IntegratorOutMin=[]  IntegratorOutMax=[]  FilterOutMin=[]  FilterOutMax=[]  SumI1OutMin=[]  SumI1OutMax=[]  SumI2OutMin=[]  SumI2OutMax=[]  SumI3OutMin=[]  SumI3OutMax=[]  SumI4OutMin=[]  SumI4OutMax=[]  SumDOutMin=[]  SumDOutMax=[]  DifferentiatorOutMin=[]  DifferentiatorOutMax=[]  FilterDiffOutCoefMin=[]  FilterDiffOutCoefMax=[]  ReciprocalOutMin=[]  ReciprocalOutMax=[]  SumDenOutMin=[]  SumDenOutMax=[]  SumNumOutMin=[]  SumNumOutMax=[]  DivideOutMin=[]  DivideOutMax=[]  UdiffTsProdOutMin=[]  UdiffTsProdOutMax=[]  NTsProdOutMin=[]  NTsProdOutMax=[]  UintegralTsProdOutMin=[]  UintegralTsProdOutMax=[]  UngainTsProdOutMin=[]  UngainTsProdOutMax=[]  ClampingZeroOutDataTypeStr=Inherit: Inherit via back propagation  ClampingZeroOutMin=[]  ClampingZeroOutMax=[]  FilterDenConstantOutDataTypeStr=Inherit: Inherit via back propagation  FilterDenConstantOutMin=[]  FilterDenConstantOutMax=[]  PCopyOutDataTypeStr=Inherit: Inherit via back propagation  PCopyOutMin=[]  PCopyOutMax=[]  NCopyOutDataTypeStr=Inherit: Inherit via back propagation  NCopyOutMin=[]  NCopyOutMax=[]  IntegratorContinuousStateAttributes=''  IntegratorStateMustResolveToSignalObject=off  IntegratorRTWStateStorageClass=Auto  FilterContinuousStateAttributes=''  FilterStateMustResolveToSignalObject=off  FilterRTWStateStorageClass=Auto  ParallelPVariant=InternalParameters  IdealPVariant=Disabled  IVariant=InternalParameters  DVariant=InternalParameters  IntegratorVariant=Continuous  SatVariant=Disabled  AWVariant=Passthrough  PCopyVariant=Disabled  TRVariant=Disabled  FdbkBlocksVariant=Forward  IdealPFdbkVariant=Disabled  SatFdbkVariant=Disabled  DerivativeFilterVariant=ContFilter  NVariant=InternalParameters  NCopyVariant=Disabled  FilterICVariant=InternalICsFilter  IntegratorICVariant=InternalICs  ExternalResetVariant=Disabled  TRSumVariant=Passthrough  SumFdbkVariant=Disabled  SumVariant=Sum_PID  TsampFilterVariant=InternalTs  TsampNgainVariant=Passthrough  TsampIntegralVariant=Disabled_SignalSpec  ExternalSaturationOutDataTypeStr=Inherit: Same as second input  DerivativeSourceVariant=ErrorSignal  PreIntVariant=InternalPreInt
  dele : Outport
  debug : Outport  Port=2
  wires:
  Constant/1 -> debug/1
  h_error/1 -> Try 1/1
  Try 1/1 -> dele/1

== system 6DoF_V8_2024a_FULLY_WORKING_FG/Aircraft_Dynamics/Aerodynamics/Aero Forces and Moments/Aerodynamic Forces ==
  CD : Inport
  CY : Inport  Port=2
  CL : Inport  Port=3
  Wind Para : Inport  Port=4
  dyn(q) : Inport  Port=5
  Body to Wind : Subsystem
  Demux : Demux  Outputs=3
      settings: DisplayOption=none
  Gain : Gain  Gain=-1  SaturateOnIntegerOverflow=on  OutDataTypeStr=Inherit: Same as input  ParamDataTypeStr=Inherit: Same as input
  Gain1 : Gain  Gain=-1  SaturateOnIntegerOverflow=on  OutDataTypeStr=Inherit: Same as input  ParamDataTypeStr=Inherit: Same as input
  Gain2 : Gain  Gain=sw  SaturateOnIntegerOverflow=on  OutDataTypeStr=Inherit: Same as input  ParamDataTypeStr=Inherit: Same as input
  Math Function : Math  Operator=transpose  SignedPower=on
  Mux : Mux  Inputs=3
  Product : Product  SaturateOnIntegerOverflow=on  OutDataTypeStr=Inherit: Same as first input
  Product1 : Product  Multiplication=Matrix(*)  SaturateOnIntegerOverflow=on  OutDataTypeStr=Inherit: Same as first input
  Terminator : Terminator
  FaeroBody : Outport
  wires:
  Gain/1 -> Mux/1
  Gain1/1 -> Mux/3
  Mux/1 -> Product/1
  Gain2/1 -> Product/2
  CD/1 -> Gain/1
  CY/1 -> Mux/2
  CL/1 -> Gain1/1
  dyn(q)/1 -> Gain2/1
  Wind Para/1 -> Demux/1
  Demux/1 -> Terminator/1
  Body to Wind/1(Smatrix) -> Math Function/1
  Math Function/1 -> Product1/1
  Product/1 -> Product1/2
  Product1/1 -> FaeroBody/1
  Demux/2 -> Body to Wind/1(Alpha)
  Demux/3 -> Body to Wind/2(Beta)

== system 6DoF_V8_2024a_FULLY_WORKING_FG/Aircraft_Dynamics/Aerodynamics/Aero Forces and Moments/Aerodynamic Moments ==
  dyn(q) : Inport
  Croll : Inport  Port=2
  CM : Inport  Port=3
  CN : Inport  Port=4
  Mux : Mux  Inputs=2
  Mux1 : Mux  Inputs=2
  Mux2 : Mux  Inputs=2
  Mux3 : Mux  Inputs=3
  Pitch : Fcn  Expr=u[1] * sw * cbar * u[2]
  Roll : Fcn  Expr=u[1] * sw * b * u[2]
  Yaw : Fcn  Expr=u[1] * sw * b * u[2]
  Maero : Outport
  wires:
  Mux/1 -> Roll/1
  Mux1/1 -> Pitch/1
  Mux2/1 -> Yaw/1
  Pitch/1 -> Mux3/2
  Roll/1 -> Mux3/1
  Yaw/1 -> Mux3/3
  dyn(q)/1 -> Mux/1, Mux1/1, Mux2/1
  Croll/1 -> Mux/2
  CM/1 -> Mux1/2
  CN/1 -> Mux2/2
  Mux3/1 -> Maero/1

== system 6DoF_V8_2024a_FULLY_WORKING_FG/Aircraft_Dynamics/Aerodynamics/CD/Get Alpha ==
  windPar : Inport
  "   " : Terminator
  "   1" : Terminator
  Demux : Demux  Outputs=3
      settings: DisplayOption=none
  Alpha : Outport
  wires:
  Demux/1 -> "   1"/1
  Demux/3 -> "   "/1
  windPar/1 -> Demux/1
  Demux/2 -> Alpha/1

== system 6DoF_V8_2024a_FULLY_WORKING_FG/Aircraft_Dynamics/Equations of motion numerical integration /Kinematic Equiations/2pi Bound ==
  In : Inport
  2pi : Constant  Value=2*pi
  Math Function : Math  Operator=mod  SignedPower=on
  Out : Outport
  wires:
  Math Function/1 -> Out/1
  2pi/1 -> Math Function/2
  In/1 -> Math Function/1

== system 6DoF_V8_2024a_FULLY_WORKING_FG/Aircraft_Dynamics/Equations of motion numerical integration /Kinematic Equiations/pi Bound ==
  In : Inport
  2pi : Constant  Value=2*pi
  Math Function : Math  Operator=mod  SignedPower=on
  Sum1 : Sum  Inputs=|+-  InputSameDT=on  SaturateOnIntegerOverflow=on  OutDataTypeStr=Inherit: Same as first input
  Sum2 : Sum  Inputs=|++  InputSameDT=on  SaturateOnIntegerOverflow=on  OutDataTypeStr=Inherit: Same as first input
  pi : Constant  Value=pi
  Out : Outport
  wires:
  Sum1/1 -> Out/1
  pi/1 -> Sum1/2, Sum2/2
  Sum2/1 -> Math Function/1
  In/1 -> Sum2/1
  2pi/1 -> Math Function/2
  Math Function/1 -> Sum1/1

== system 6DoF_V8_2024a_FULLY_WORKING_FG/Aircraft_Dynamics/Equations of motion numerical integration /Kinematic Equiations/pi Bound1 ==
  In : Inport
  2pi : Constant  Value=2*pi
  Math Function : Math  Operator=mod  SignedPower=on
  Sum1 : Sum  Inputs=|+-  InputSameDT=on  SaturateOnIntegerOverflow=on  OutDataTypeStr=Inherit: Same as first input
  Sum2 : Sum  Inputs=|++  InputSameDT=on  SaturateOnIntegerOverflow=on  OutDataTypeStr=Inherit: Same as first input
  pi : Constant  Value=pi
  Out : Outport
  wires:
  Sum1/1 -> Out/1
  pi/1 -> Sum1/2, Sum2/2
  Sum2/1 -> Math Function/1
  In/1 -> Sum2/1
  2pi/1 -> Math Function/2
  Math Function/1 -> Sum1/1

== system 6DoF_V8_2024a_FULLY_WORKING_FG/Aircraft_Dynamics/Equations of motion numerical integration /Moment Equations/Inertia Coefs ==
  note: Jx,Jy,Jz,Jxz
  note: Inertia Coefficeents
      | Page 80 Stevens and Lewis
  Inertia : Inport
  Mux : Mux  Inputs=9
  c1 : Fcn  Expr=((u[2]-u[3])*u[3] - u[4]^2)/(u[1]*u[3]-u[4]^2)
  c2 : Fcn  Expr=((u[1]-u[2]+u[3])*u[4])/(u[1]*u[3]-u[4]^2)
  c3 : Fcn  Expr=u[3]/(u[1]*u[3]-u[4]^2)
  c4 : Fcn  Expr=u[4]/(u[1]*u[3]-u[4]^2)
  c5 : Fcn  Expr=(u[3]-u[1])/u[2]
  c6 : Fcn  Expr=u[4]/u[2]
  c7 : Fcn  Expr=1/u[2]
  c8 : Fcn  Expr=(u[1]*(u[1]-u[2])+u[4]^2)/(u[1]*u[3]-u[4]^2)
  c9 : Fcn  Expr=u[1]/(u[1]*u[3]-u[4]^2)
  Iner Coef : Outport
  wires:
  Inertia/1 -> c1/1, c2/1, c3/1, c4/1, c5/1, c6/1, c7/1, c9/1, c8/1
  c1/1 -> Mux/1
  c2/1 -> Mux/2
  c3/1 -> Mux/3
  c4/1 -> Mux/4
  c5/1 -> Mux/5
  c6/1 -> Mux/6
  c7/1 -> Mux/7
  c8/1 -> Mux/8
  c9/1 -> Mux/9
  Mux/1 -> Iner Coef/1

== system 6DoF_V8_2024a_FULLY_WORKING_FG/Aircraft_Dynamics/Aerodynamics/Aero Forces and Moments/Aerodynamic Forces/Body to Wind ==
  note: This transforms any arbitrary vector from body axis to wind axis.
      | Page 63  Stevens and Lewis
  Alpha : Inport
  Beta : Inport  Port=2
  -ca sb : Fcn  Expr=-1 * cos(u[1]) * sin(u[2])
  -sa : Fcn  Expr=-1 * sin(u[1])
  -sa sb : Fcn  Expr="-1 * sin(u[1])  * sin(u[2])"
  Fcn8 : Fcn  Expr=cos(u[1])
  Matrix Concatenation : Concatenate  NumInputs=3  Mode=Multidimensional array
  Matrix Concatenation1 : Concatenate  NumInputs=3  Mode=Multidimensional array
  Matrix Concatenation2 : Concatenate  NumInputs=3  Mode=Multidimensional array  ConcatenateDimension=2
  Matrix Concatenation3 : Concatenate  NumInputs=3  Mode=Multidimensional array
  Mux1 : Mux  Inputs=2
  ca cb : Fcn  Expr="cos(u[1]) *  cos(u[2])"
  cb : Fcn  Expr=cos(u[2])
  sa cb : Fcn  Expr=sin(u[1]) * cos(u[2])
  sb : Fcn  Expr=sin(u[2])
  zero : Fcn  Expr=u[1] * 0
  Smatrix : Outport
  wires:
  Matrix Concatenation/1 -> Matrix Concatenation2/1
  Matrix Concatenation1/1 -> Matrix Concatenation2/2
  Matrix Concatenation3/1 -> Matrix Concatenation2/3
  -ca sb/1 -> Matrix Concatenation/2
  ca cb/1 -> Matrix Concatenation/1
  -sa/1 -> Matrix Concatenation/3
  zero/1 -> Matrix Concatenation1/3
  sb/1 -> Matrix Concatenation1/1
  cb/1 -> Matrix Concatenation1/2
  sa cb/1 -> Matrix Concatenation3/1
  -sa sb/1 -> Matrix Concatenation3/2
  Fcn8/1 -> Matrix Concatenation3/3
  Mux1/1 -> ca cb/1, -ca sb/1, -sa/1, sb/1, cb/1, zero/1, sa cb/1, -sa sb/1, Fcn8/1
  Alpha/1 -> Mux1/1
  Beta/1 -> Mux1/2
  Matrix Concatenation2/1 -> Smatrix/1

== matlab function 6DoF_V8_2024a_FULLY_WORKING_FG/Subsystem1/MATLAB Function ==
  data: N input; Lat output; r input
function Lat = fcn(N,r)

Lat = 90-(acos(N/r))*(180/pi);

== matlab function 6DoF_V8_2024a_FULLY_WORKING_FG/Subsystem1/MATLAB Function1 ==
  data: r input; E input; Long output
function Long = fcn(r,E)

Long = (atan(E/r))*(180/pi);
